simulink model "FIR"  (R2020b)
settings: Solver=VariableStepAuto  StartTime=0.0  StopTime=10.0  RelTol=1e-3
settings Model: Creator=Puru Gawande  LastModifiedBy=Puru Gawande

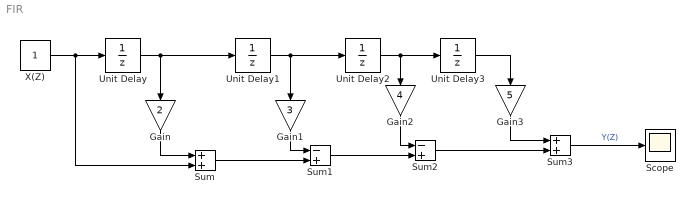
== system FIR ==
  Gain : Gain  Gain=2
  Gain1 : Gain  Gain=3
  Gain2 : Gain  Gain=4
  Gain3 : Gain  Gain=5
  Scope : Scope
  Sum : Sum
  Sum1 : Sum  Inputs=-+
  Sum2 : Sum  Inputs=-+
  Sum3 : Sum
  Unit Delay{,1..3} (4 alike) : UnitDelay  SampleTime=-1  HasFrameUpgradeWarning=on
  X(Z) : Constant
  wires:
  X(Z)/1 -> Unit Delay/1, Sum/2
  Unit Delay/1 -> Gain/1, Unit Delay1/1
  Sum/1 -> Sum1/2
  Unit Delay1/1 -> Gain1/1, Unit Delay2/1
  Unit Delay2/1 -> Unit Delay3/1, Gain2/1
  Sum1/1 -> Sum2/2
  Gain/1 -> Sum/1
  Gain1/1 -> Sum1/1
  Gain2/1 -> Sum2/1
  Sum2/1 -> Sum3/2
  Gain3/1 -> Sum3/1
  Unit Delay3/1 -> Gain3/1
  Sum3/1 -> Scope/1  "Y(Z)"
